simulink model "ZAD1_2_Model"  (R2018a)
settings: Solver=ode45  StartTime=0.0  StopTime=tend  MaxStep=Tp  RelTol=1e-3
undefined symbols (not defined in the file or in its folder): initConditionsAcc, initConditionsVel, Kp, Kv, omega1, omega2, Qd01, Qd02, Qd1, Qd11, Qd12, Qd1const, Qd2, Qd21, Qd22, Qd2const, Qd31, Qd32
libraries: simulink x3
settings Model: Creator=szymon  LastModifiedBy=szymon

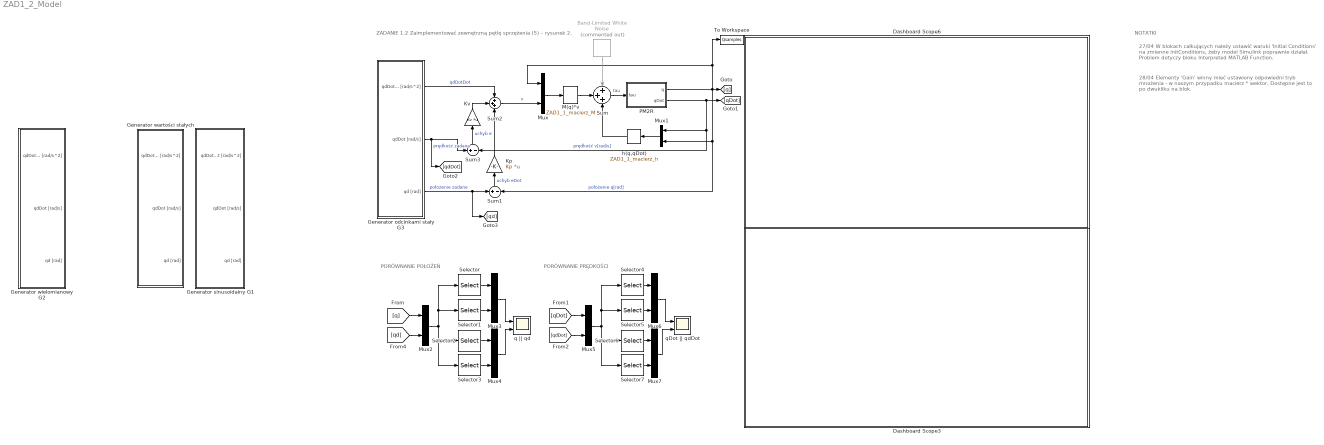
== system ZAD1_2_Model ==
  note: PORÓWNANIE POŁOŻEŃ
  note: NOTATKI
  note: ZADANIE 1.2
      |  Zaimplementować zewnętrzną pętlę sprzężenia (5) – rysunek 2.
  note: 27/04 W blokach całkujących należy ustawić waruki
      | 'Initial Conditions' na zmienne initConditions, żeby model
      | Simulink poprawnie działał. Problem dotyczy bloku
      | Interpreted MATLAB Function.
  note: 28/04 Elementy 'Gain' winny mieć ustawiony odpowiedni tryb
      | mnożenia - w naszym przypadku macierz * wektor.
      | Dostępne jest to po dwukliku na blok.
  note: PORÓWNANIE PRĘDKOŚCI
  Band-Limited White Noise : simulink/Sources/Band-Limited White Noise  Commented=on  Cov=[0.1]  Ts=0.1  seed=[23341]
  Dashboard Scope3 : Subsystem  DialogController=hmiCreateDDGDialog  IsWebBlock=on  mask(MWDashboardBlock){webBlockId=7e31f546-b89a-4450-b53f-669fe20aafff, webBlockType=sdiscope, ShowInitialText=on, HMISrcModelName=ZAD1_2_Model}
      mask prompts: webBlockId "WebBlock Id"; webBlockType "WebBlock Type"; HMISrcModelName "Source Model"
      mask help: SimulinkHMI:dialogs:HMIScopeDialogDesc
      mask Help: helpview([docroot '/mapfiles/simulink.map'], 'hmi_scope')
      mask Display:
      | if strcmp(get_param(bdroot(gcb),'BlockDiagramType'), 'library')
      |     image([(matlabroot) '/toolbox/simulink/hmi/icons/DashboardScope.png']);
      | end
  Dashboard Scope6 : Subsystem  DialogController=hmiCreateDDGDialog  IsWebBlock=on  mask(MWDashboardBlock){webBlockId=060137c1-44cd-42f9-89eb-7b1da18c6d2d, webBlockType=sdiscope, ShowInitialText=on, HMISrcModelName=ZAD1_2_Model}
      mask prompts: webBlockId "WebBlock Id"; webBlockType "WebBlock Type"; HMISrcModelName "Source Model"
      mask help: SimulinkHMI:dialogs:HMIScopeDialogDesc
      mask Help: helpview([docroot '/mapfiles/simulink.map'], 'hmi_scope')
      mask Display:
      | if strcmp(get_param(bdroot(gcb),'BlockDiagramType'), 'library')
      |     image([(matlabroot) '/toolbox/simulink/hmi/icons/DashboardScope.png']);
      | end
  "Generator odcinkami stały G3 " : Subsystem
  Generator sinusoidalny G1 : Subsystem
  Generator wielomianowy G2 : Subsystem
  Generator wartości stałych : Subsystem
  Kp : Gain  Gain=Kp  Multiplication=Matrix(K*u)
  Kv : Gain  Gain=Kv  Multiplication=Matrix(K*u)
  M(q)*v : MATLABFcn  MATLABFcn=ZAD1_1_macierz_M
  Mux{,1..7} (8 alike) : Mux  Inputs=2
  PM2R : Subsystem
  Selector : Selector  InputPortWidth=4  IndexOptions=Index vector (dialog)  Indices=[1]  OutputSizes=1
  Selector1 : Selector  InputPortWidth=4  IndexOptions=Index vector (dialog)  Indices=[3]  OutputSizes=1
  Selector2 : Selector  InputPortWidth=4  IndexOptions=Index vector (dialog)  Indices=[2]  OutputSizes=1
  Selector3 : Selector  InputPortWidth=4  IndexOptions=Index vector (dialog)  Indices=[4]  OutputSizes=1
  Selector4 : Selector  InputPortWidth=4  IndexOptions=Index vector (dialog)  Indices=[1]  OutputSizes=1
  Selector5 : Selector  InputPortWidth=4  IndexOptions=Index vector (dialog)  Indices=[3]  OutputSizes=1
  Selector6 : Selector  InputPortWidth=4  IndexOptions=Index vector (dialog)  Indices=[2]  OutputSizes=1
  Selector7 : Selector  InputPortWidth=4  IndexOptions=Index vector (dialog)  Indices=[4]  OutputSizes=1
  Sum : Sum  Inputs=+++
  Sum1 : Sum  Inputs=+-
  Sum2 : Sum  Inputs=+++
  Sum3 : Sum  Inputs=+-
  To Workspace : ToWorkspace  VariableName=Qsamples  SampleTime=-1
  h(q,qDot) : MATLABFcn  MATLABFcn=ZAD1_1_macierz_h
  q || qd : Scope  NumInputPorts=2
  qDot || qdDot : Scope  NumInputPorts=2
  wires:
  Mux/1 -> M(q)*v/1
  Mux1/1 -> h(q,qDot)/1
  h(q,qDot)/1 -> Sum/3
  M(q)*v/1 -> Sum/2
  Sum/1 -> PM2R/1(tau)  "tau"
  PM2R/2(qDot) -> [qDot], Mux1/1, Sum3/2  "prędkość v[rad/s]"
  "Generator odcinkami stały G3 "/3(qd [rad]) -> [qd], Sum1/1  "położenie zadane"
  Sum1/1 -> Kp/1  "uchyb eDot"
  Sum2/1 -> Mux/2  "v"
  "Generator odcinkami stały G3 "/1(qdDotDot [rad/s^2]) -> Sum2/1  "qdDotDot"
  "Generator odcinkami stały G3 "/2(qdDot [rad/s]) -> Sum3/1, [qdDot]  "prędkość zadana"
  Kv/1 -> Sum2/2
  Kp/1 -> Sum2/3
  Sum3/1 -> Kv/1  "uchyb e"
  PM2R/1(q) -> [q], Mux/1, To Workspace/1, Mux1/2, Sum1/2  "położenie q[rad]"
  Band-Limited White Noise/1 -> Sum/1
  [q] -> Mux2/1
  [qd] -> Mux2/2
  Selector/1 -> Mux3/1
  Selector1/1 -> Mux3/2
  Selector2/1 -> Mux4/1
  Selector3/1 -> Mux4/2
  Mux2/1 -> Selector3/1, Selector2/1, Selector1/1, Selector/1
  Mux3/1 -> q || qd/1
  Mux4/1 -> q || qd/2
  Selector6/1 -> Mux7/1
  Mux6/1 -> qDot || qdDot/1
  Mux7/1 -> qDot || qdDot/2
  Selector7/1 -> Mux7/2
  [qDot] -> Mux5/1
  Selector5/1 -> Mux6/2
  [qdDot] -> Mux5/2
  Selector4/1 -> Mux6/1
  Mux5/1 -> Selector7/1, Selector6/1, Selector5/1, Selector4/1

== system ZAD1_2_Model/Dashboard Scope3 ==

== system ZAD1_2_Model/Dashboard Scope6 ==

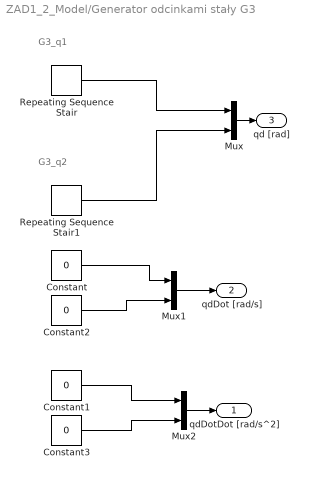
== system ZAD1_2_Model/Generator odcinkami stały G3  ==
  note: G3_q2
  note: G3_q1
  Constant{,1..3} (4 alike) : Constant  Value=0
  Mux : Mux  Inputs=2
  Mux1 : Mux  Inputs=2
  Mux2 : Mux  Inputs=2
  Repeating Sequence Stair : simulink/Sources/Repeating Sequence Stair  OutValues=[Qd1const 0].'  tsamp=Ta  OutMin=[]  OutMax=[]  OutDataTypeStr=double  OutputDataTypeScalingMode=double  OutDataType=fixdt(0,8)  ConRadixGroup=Best Precision: Vector-wise  OutScaling=2^-12
  Repeating Sequence Stair1 : simulink/Sources/Repeating Sequence Stair  OutValues=[Qd2const 0].'  tsamp=Tb  OutMin=[]  OutMax=[]  OutDataTypeStr=double  OutputDataTypeScalingMode=double  OutDataType=fixdt(0,8)  ConRadixGroup=Best Precision: Vector-wise  OutScaling=2^-12
  qdDotDot [rad/s^2] : Outport
  qdDot [rad/s] : Outport  Port=2
  qd [rad] : Outport  Port=3
  wires:
  Constant/1 -> Mux1/1
  Repeating Sequence Stair1/1 -> Mux/2
  Repeating Sequence Stair/1 -> Mux/1
  Mux/1 -> qd [rad]/1
  Constant1/1 -> Mux2/1
  Constant2/1 -> Mux1/2
  Constant3/1 -> Mux2/2
  Mux2/1 -> qdDotDot [rad/s^2]/1
  Mux1/1 -> qdDot [rad/s]/1

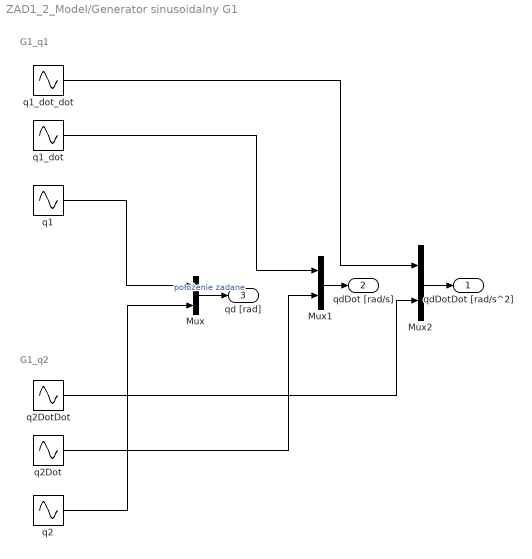
== system ZAD1_2_Model/Generator sinusoidalny G1 ==
  note: G1_q2
  note: G1_q1
  Mux : Mux  Inputs=2
  Mux1 : Mux  Inputs=2
  Mux2 : Mux  Inputs=2
  "q1 " : Sin  Amplitude=Qd1  Frequency=omega1  SampleTime=0
  q1_dot : Sin  Amplitude=omega1*Qd1  Frequency=omega1  Phase=pi/2  SampleTime=0
  "q1_dot_dot " : Sin  Amplitude=-omega1^2*Qd1  Frequency=omega1  SampleTime=0
  q2 : Sin  Amplitude=Qd2  Frequency=omega2  SampleTime=0
  q2Dot : Sin  Amplitude=omega2*Qd2  Frequency=omega2  Phase=pi/2  SampleTime=0
  "q2DotDot " : Sin  Amplitude=-omega2^2*Qd2  Frequency=omega2  SampleTime=0
  qdDotDot [rad/s^2] : Outport
  qdDot [rad/s] : Outport  Port=2
  qd [rad] : Outport  Port=3
  wires:
  Mux1/1 -> qdDot [rad/s]/1
  Mux2/1 -> qdDotDot [rad/s^2]/1
  "q1_dot_dot "/1 -> Mux2/1
  "q2DotDot "/1 -> Mux2/2
  q2Dot/1 -> Mux1/2
  q1_dot/1 -> Mux1/1
  q2/1 -> Mux/2
  "q1 "/1 -> Mux/1
  Mux/1 -> qd [rad]/1  "położenie zadane"

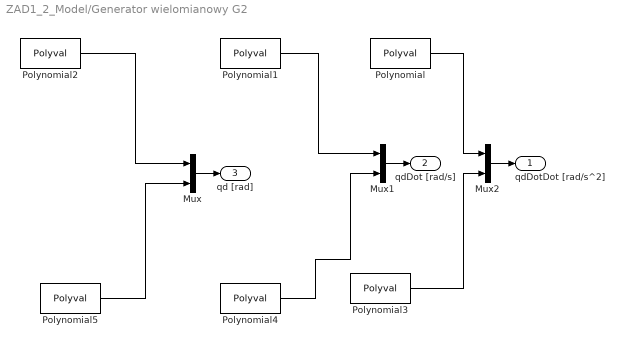
== system ZAD1_2_Model/Generator wielomianowy G2 ==
  Mux : Mux  Inputs=2
  Mux1 : Mux  Inputs=2
  Mux2 : Mux  Inputs=2
  Polynomial : Polyval  Coefs=[6*Qd31*t, 2*Qd21]
  Polynomial1 : Polyval  Coefs=[3*Qd31*t.^2, 2*Qd21*t, Qd11]
  Polynomial2 : Polyval  Coefs=[Qd31*t.^3, Qd21*t.^2, Qd11*t, Qd01]
  Polynomial3 : Polyval  Coefs=[6*Qd32*t, 2*Qd22]
  Polynomial4 : Polyval  Coefs=[3*Qd32*t.^2, 2*Qd22*t, Qd12]
  Polynomial5 : Polyval  Coefs=[Qd32*t.^3, Qd22*t.^2, Qd12*t, Qd02]
  qdDotDot [rad/s^2] : Outport
  qdDot [rad/s] : Outport  Port=2
  qd [rad] : Outport  Port=3
  wires:
  Polynomial/1 -> Mux2/1
  Polynomial1/1 -> Mux1/1
  Polynomial2/1 -> Mux/1
  Polynomial3/1 -> Mux2/2
  Polynomial5/1 -> Mux/2
  Polynomial4/1 -> Mux1/2
  Mux/1 -> qd [rad]/1
  Mux1/1 -> qdDot [rad/s]/1
  Mux2/1 -> qdDotDot [rad/s^2]/1

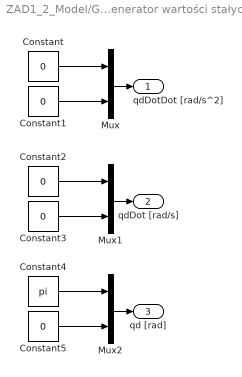
== system ZAD1_2_Model/Generator wartości stałych ==
  Constant{,1..3,5} (5 alike) : Constant  Value=0
  Constant4 : Constant  Value=pi
  Mux : Mux  Inputs=2
  Mux1 : Mux  Inputs=2
  Mux2 : Mux  Inputs=2
  qdDotDot [rad/s^2] : Outport
  qdDot [rad/s] : Outport  Port=2
  qd [rad] : Outport  Port=3
  wires:
  Constant/1 -> Mux/1
  Mux/1 -> qdDotDot [rad/s^2]/1
  Constant1/1 -> Mux/2
  Constant2/1 -> Mux1/1
  Constant3/1 -> Mux1/2
  Mux1/1 -> qdDot [rad/s]/1
  Constant4/1 -> Mux2/1
  Constant5/1 -> Mux2/2
  Mux2/1 -> qd [rad]/1

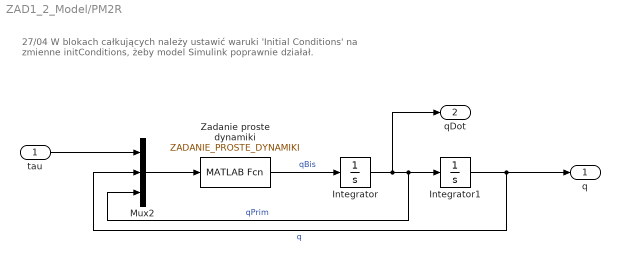
== system ZAD1_2_Model/PM2R ==
  note: 27/04 W blokach całkujących należy ustawić waruki 'Initial Conditions' na
      | zmienne initConditions, żeby model Simulink poprawnie działał.
  tau : Inport
  Integrator : Integrator  InitialCondition=initConditionsAcc
  Integrator1 : Integrator  InitialCondition=initConditionsVel
  Mux2 : Mux  Inputs=3
  Zadanie proste dynamiki : MATLABFcn  MATLABFcn=ZADANIE_PROSTE_DYNAMIKI
  q : Outport
  qDot : Outport  Port=2
  wires:
  Zadanie proste dynamiki/1 -> Integrator/1  "qBis"
  Integrator/1 -> qDot/1, Mux2/3, Integrator1/1  "qPrim"
  Integrator1/1 -> q/1, Mux2/2  "q"
  tau/1 -> Mux2/1
  Mux2/1 -> Zadanie proste dynamiki/1
